simulink model "Intgr1"  (Simulink 8.5)
settings: Solver=ode1  SolverMode=SingleTasking  StartTime=0.0  StopTime=32  FixedStep=Ts  RelTol=1e-3
values from neighbouring files (symbols this model uses):
  k1 = 0.1    [init.m]
  k2 = 0.1    [init.m]
  kf = 0.1    [init.m]
  Ts = 1    [init.m]
undefined symbols (not defined in the file or in its folder): j
undefined symbols (not defined in the file): klp
settings Model: Creator=martin  LastModifiedBy=martin
settings DataIOCC: SignalLoggingSaveFormat=Dataset
settings OptimizationCC: ExpressionDepthLimit=128
settings DebuggingCC: UnderspecifiedInitializationDetection=Simplified  MergeDetectMultiDrivingBlocksExec=error  FcnCallInpInsideContextMsg=EnableAllAsError  StateNameClashWarn=none
settings GRTTargetCC: CombineOutputUpdateFcns=on  GRTInterface=off

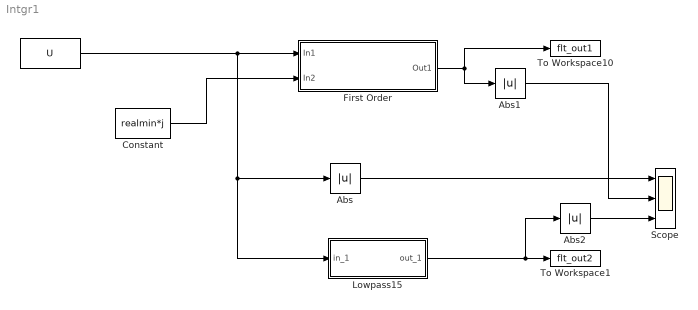
== system Intgr1 ==
  " " : FromWorkspace  VariableName=U  SampleTime=Ts
  Abs : Abs
  Abs1 : Abs
  Abs2 : Abs
  Constant : Constant  Value=realmin*j
  First Order : Subsystem  mask{k1=k1, k2=k2, kf=kf}
      mask Display:
      | disp(sprintf('k1r = %0.6g k1r = %0.6g\nk2r = %0.6g k2i = %0.6g\nkfr = %0.6g kfi = %0.6g', ...
      |     real(k1), imag(k1), real(k2), imag(k2), real(kf), imag(kf)));
  Lowpass15 : Subsystem  mask(1'st Order Lowpass){k1=klp, Ts=Ts}
      mask help: 3'rd Order Low-Pass
      mask Help: f-3dB = k/(2*pi)
      mask Display: disp('1st Order Lowpass')
  Scope : Scope  NumInputPorts=3
      settings: TimeRange=511  YMin=0~0~0  YMax=1~0.1~0.25  MaxDataPoints=2000000  SampleInput=on  SampleTime=Ts
  To Workspace1 : ToWorkspace  VariableName=flt_out2  SampleTime=-1
      settings: MaxDataPoints=128*16 - 1
  To Workspace10 : ToWorkspace  VariableName=flt_out1  SampleTime=-1
      settings: MaxDataPoints=128*16 - 1
  wires:
  " "/1 -> Abs/1, Lowpass15/1(in_1), First Order/1(In1)
  First Order/1(Out1) -> Abs1/1, To Workspace10/1
  Lowpass15/1(out_1) -> Abs2/1, To Workspace1/1
  Constant/1 -> First Order/2(In2)
  Abs/1 -> Scope/1
  Abs1/1 -> Scope/2
  Abs2/1 -> Scope/3

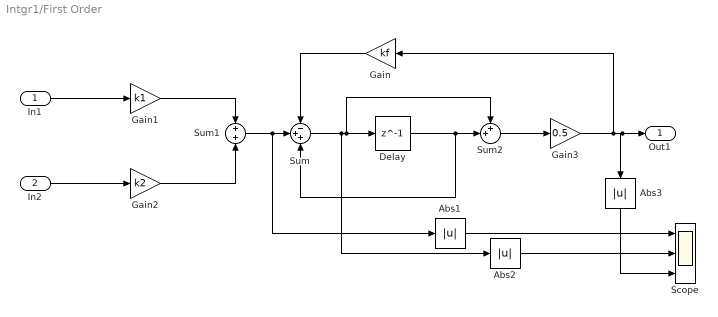
== system Intgr1/First Order ==
  In1 : Inport
      settings: SignalType=complex
  In2 : Inport  Port=2
  Abs1 : Abs
  Abs2 : Abs
  Abs3 : Abs
  Delay : Delay  DelayLength=1
  Gain : Gain  Gain=kf
  Gain1 : Gain  Gain=k1
  Gain2 : Gain  Gain=k2
  Gain3 : Gain  Gain=0.5
  Scope : Scope  NumInputPorts=3
      settings: TimeRange=511  YMin=0~0~0  YMax=1~0.1~0.25  MaxDataPoints=2000000  SampleInput=on  SampleTime=Ts
  Sum : Sum  Inputs=-++
  Sum1 : Sum  Inputs=+|+
  Sum2 : Sum  Inputs=++|
  Out1 : Outport
      settings: SignalType=complex
  wires:
  Gain/1 -> Sum/1
  In1/1 -> Gain1/1
  Sum1/1 -> Abs1/1, Sum/2
  In2/1 -> Gain2/1
  Sum/1 -> Abs2/1, Sum2/1, Delay/1
  Gain2/1 -> Sum1/2
  Gain1/1 -> Sum1/1
  Delay/1 -> Sum2/2, Sum/3
  Sum2/1 -> Gain3/1
  Gain3/1 -> Gain/1, Abs3/1, Out1/1
  Abs1/1 -> Scope/1
  Abs2/1 -> Scope/2
  Abs3/1 -> Scope/3

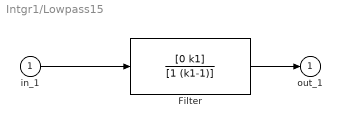
== system Intgr1/Lowpass15 ==
  in_1 : Inport
  Filter : DiscreteFilter  Numerator=[0 k1]  Denominator=[1 (k1-1)]  SampleTime=Ts
  out_1 : Outport  InitialOutput=0
  wires:
  Filter/1 -> out_1/1
  in_1/1 -> Filter/1
